simulink model "threesinglesourcefull"  (R2013b)
settings: Solver=ode45  StartTime=0.0  StopTime=0.04  RelTol=1e-3
undefined symbols (not defined in the file): alpha
libraries: powerlib x28
settings Model: Creator=SAI KUMAR  LastModifiedBy=SAI KUMAR

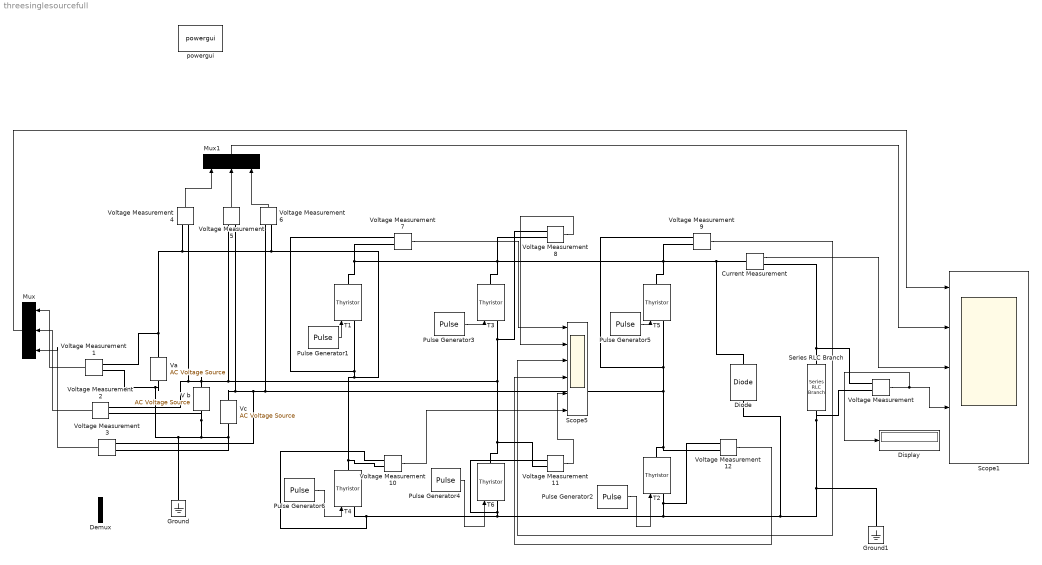
== system threesinglesourcefull ==
  Current Measurement : powerlib/Measurements/Current Measurement  PhasorSimulation=off  OutputType=Complex  PSBequivalent=0
  Demux : Demux  Outputs=2
  Diode : powerlib/Power Electronics/Diode  Ron=0.001  Lon=0  Vf=0.8  IC=0  UseSnubber=off  Rs=500  Cs=250e-9  Measurements=off
  Display : Display
  Ground : powerlib/Elements/Ground  LConnTagsString=a
  Ground1 : powerlib/Elements/Ground  LConnTagsString=a
  Mux : Mux  Inputs=3
  Mux1 : Mux  Inputs=3
  Pulse Generator1 : DiscretePulseGenerator  PulseType=Time based  Amplitude=5  Period=0.02  PhaseDelay=((0.02/360)*alpha)+((0.02/360)*30)
  Pulse Generator2 : DiscretePulseGenerator  PulseType=Time based  Amplitude=5  Period=0.02  PhaseDelay=((0.02/360)*alpha)+((0.02/360)*90)
  Pulse Generator3 : DiscretePulseGenerator  PulseType=Time based  Amplitude=5  Period=0.02  PhaseDelay=((0.02/360)*150)+((0.02/360)*alpha)
  Pulse Generator4 : DiscretePulseGenerator  PulseType=Time based  Amplitude=5  Period=0.02  PhaseDelay=((0.02/360)*alpha)+((0.02/360)*330)
  Pulse Generator5 : DiscretePulseGenerator  PulseType=Time based  Amplitude=5  Period=0.02  PhaseDelay=((0.02/360)*270)+((0.02/360)*alpha)
  Pulse Generator6 : DiscretePulseGenerator  PulseType=Time based  Amplitude=5  Period=0.02  PhaseDelay=((0.02/360)*210)+((0.02/360)*alpha)
  Scope1 : Scope  NumInputPorts=5
      settings: TimeRange=5  YMin=5~-5~-5~-5~-5  YMax=85~5~5~5~5  SampleInput=on
  Scope5 : Scope  NumInputPorts=6
      settings: TimeRange=5  YMin=5~-5~-5~-5~-5~-5  YMax=85~5~5~5~5~5  SampleInput=on
  Series RLC Branch : powerlib/Elements/Series RLC Branch  LConnTagsString=__new0  RConnTagsString=__new0  BranchType=R  Resistance=10  Inductance=1e-3  SetiL0=off  InitialCurrent=0  Capacitance=1e-6  Setx0=off  InitialVoltage=0  Measurements=None
  T{1..6} (6 alike) : powerlib/Power Electronics/Thyristor  Ron=0.001  Lon=0  Vf=0.8  IC=0  Rs=500  Cs=250e-9  Measurements=off
  V b : powerlib/Electrical Sources/AC Voltage Source  Amplitude=220*sqrt(2)  Phase=-120  Frequency=50  SampleTime=0  Measurements=Voltage
  Va : powerlib/Electrical Sources/AC Voltage Source  Amplitude=220*sqrt(2)  Phase=0  Frequency=50  SampleTime=0  Measurements=Voltage
  Vc : powerlib/Electrical Sources/AC Voltage Source  Amplitude=220*sqrt(2)  Phase=120  Frequency=50  SampleTime=0  Measurements=Voltage
  Voltage Measurement{,1..12} (13 alike) : powerlib/Measurements/Voltage Measurement  PhasorSimulation=off  OutputType=Complex  PSBequivalent=0
  powergui : powerlib/powergui  Priority=1  SimulationMode=Continuous  SolverType=Tustin  SampleTime=50e-6  frequency=60  SPID=off  DisableSnubberDevices=off  DisableRonSwitches=off  DisableVfSwitches=off  SwTol=0  Interpol=off  DisplayEquations=off  frequencyindice=50  Pbase=100e6  ErrMax=1e-4  Iterations=50  UnitsV=kV  UnitsW=MW  FunctionMessages=off  echomessages=off  HookPort=off  EnableUseOfTLC=off  x0status=blocks  RestoreLinks=warning  ResistiveCurrentMeasurement=off  Frange=[0:2:500]  Ylog=off  Xlog=on  ShowGrid=off  save=off  variable=ZData  ZoomFFT=off  StartTime=0.0  cycles=1  DisplayStyle=1  fundamental=60  FreqAxis=off  MaxFrequency=1000  frequencyindicesteady=1  RmsSteady=1  display=off  Ts=0  methode=off
  wires:
  Voltage Measurement1/1 -> Mux/1
  Voltage Measurement2/1 -> Mux/2
  Voltage Measurement3/1 -> Mux/3
  Mux/1 -> Scope1/1
  Pulse Generator1/1 -> T1/1
  Pulse Generator2/1 -> T2/1
  Pulse Generator3/1 -> T3/1
  Pulse Generator4/1 -> T6/1
  Pulse Generator5/1 -> T5/1
  Pulse Generator6/1 -> T4/1
  Voltage Measurement4/1 -> Mux1/1
  Voltage Measurement5/1 -> Mux1/2
  Voltage Measurement6/1 -> Mux1/3
  Voltage Measurement/1 -> Display/1, Scope1/4
  Current Measurement/1 -> Scope1/3
  Mux1/1 -> Scope1/2
  Voltage Measurement7/1 -> Scope5/1
  Voltage Measurement8/1 -> Scope5/2
  Voltage Measurement9/1 -> Scope5/3
  Voltage Measurement12/1 -> Scope5/4
  Voltage Measurement11/1 -> Scope5/5
  Voltage Measurement10/1 -> Scope5/6
  connections:
  Va/LConn1 -- Ground/LConn1 -- Voltage Measurement3/LConn2 -- Vc/LConn1 -- Voltage Measurement2/LConn2 -- V b/LConn1 -- Voltage Measurement1/LConn2
  T1/RConn1 -- Voltage Measurement7/LConn2 -- Voltage Measurement8/LConn2 -- T3/RConn1 -- Diode/RConn1 -- Current Measurement/LConn1 -- T5/RConn1 -- Voltage Measurement9/LConn2
  T4/LConn1 -- Voltage Measurement10/LConn1 -- Voltage Measurement11/LConn1 -- T6/LConn1 -- Ground1/LConn1 -- Voltage Measurement/LConn2 -- Series RLC Branch/RConn1 -- Diode/LConn1 -- Voltage Measurement12/LConn1 -- T2/LConn1
  Current Measurement/RConn1 -- Voltage Measurement/LConn1 -- Series RLC Branch/LConn1
  T1/LConn1 -- Voltage Measurement7/LConn1 -- Voltage Measurement6/LConn2 -- Voltage Measurement1/LConn1 -- Va/RConn1 -- Voltage Measurement4/LConn1 -- Voltage Measurement10/LConn2 -- T4/RConn1
  T5/LConn1 -- Voltage Measurement9/LConn1 -- Voltage Measurement6/LConn1 -- Voltage Measurement3/LConn1 -- Voltage Measurement5/LConn2 -- Vc/RConn1 -- Voltage Measurement12/LConn2 -- T2/RConn1
  T3/LConn1 -- Voltage Measurement8/LConn1 -- Voltage Measurement5/LConn1 -- Voltage Measurement4/LConn2 -- Voltage Measurement2/LConn1 -- V b/RConn1 -- Voltage Measurement11/LConn2 -- T6/RConn1
